simulink model "PV_microgrid"  (R2022b)
settings: Solver=FixedStepAuto  StartTime=0.0  StopTime=0.6  FixedStep=1e-6  RelTol=1e-3
model workspace (MAT data in the model file):
  C = 0.002
  D = 100
  GP = 1
  GQ = 1
  I1 = 100
  I2 = 50
  J = 3.5
  KQ = 0.06
  Kf = 120
  Kv = 577
  L = 2e-05
  LS = 0.003
  P1 = 0.2
  P2 = 6
  Pref = 500000
  Qref = 0
  Ts = 0.0001
  Ts_power = 1e-06
  Ug = 563.38264084
  fsw = 10000
  t0 = 0.5
  wn = 314.159265359
undefined symbols (not defined in the file): D1, Delta, DiscIntNeverNeededParam, Ion, Lithium, LL, LP, Ts_Power
libraries: spsSeriesRLCBranchLib x9, spsFirstOrderFilterLib x7, slpidlib x5, spsMeanLib x5, spsabctodq0Lib x4, spsStairGeneratorLib x4, spsThreePhaseVIMeasurementLib x3, spsThreePhaseTransformerTwoWindingsLib x2, spsThreePhaseParallelRLCLoadLib x2, spsThreePhasePISectionLineLib x2, spsBoostConverterLib x2, spsPowerPositiveSequenceLib x2
(part 1 of 2)
settings Model: SimulationMode=accelerator  Creator=刘明炜  LastModifiedBy=刘明炜

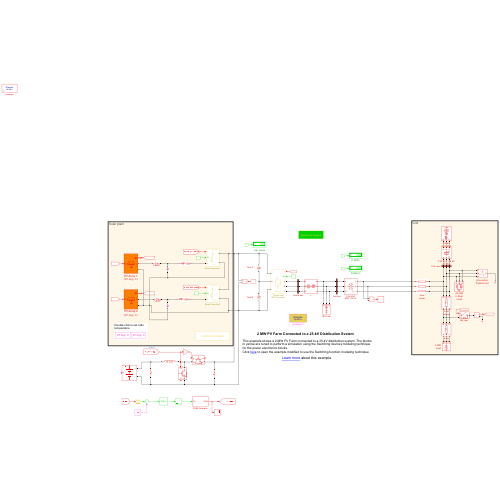
[thumbnail: Simulink's stored preview of the top-level diagram]
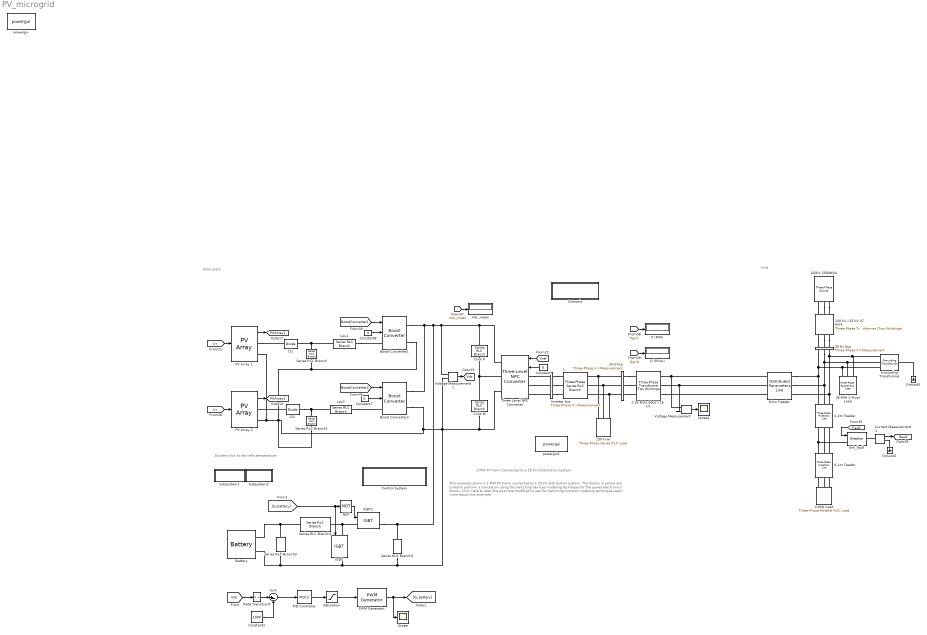
== system PV_microgrid ==
  note: Solar plant
  note: Double-click to set cells temperature
  note: This example shows a 2-MW PV Farm connected to a 25-kV distribution system. The blocks in yellow are tuned to perform a simulation using the Switching devices modeling technique for the power electronics blocks.
      | Click here to open the example modified to use the Switching function modeling technique
      |
      | Learn more about this example.
  note: 2 MW PV Farm Connected to a 25-kV Distribution System
  note: Grid
  120 kV / 25 kV 47 MVA : spsThreePhaseTransformerTwoWindingsLib/Three-Phase Transformer (Two Windings)  Winding1Connection=Yg  Winding2Connection=Delta (D1)  CoreType=Three single-phase transformers  SetSaturation=off  Hysteresis=off  DataFile='basic_model'  SetInitialFlux=off  Measurements=None  UNITS=pu  NominalPower=[47e6 50 ]  Winding1="[ 120e3  0.08/30   0.08 ]"  Winding2="[ 25e3 0.08/30  0.08]"  Rm=500  Lm=500  L0=0.5  Saturation="[ 0,0  ;  0.005,1.2  ;  1.0,1.4 ]"  InitialFluxes=[ 0.8 , -0.8 , 0.7 ]  BreakLoop=off  DiscreteSolver=Trapezoidal iterative  DataType=off  TransfoNumber=0
  120kV 2500MVA : spsThreePhaseSourceLib/Three-Phase Source  InternalConnection=Yg  VoltagePhases=off  Voltage=120e3*1.02  PhaseAngle=0  Voltage_phases=[25e3 25e3 25e3]/sqrt(3)  PhaseAngles_phases=[0 -120 +120]  Frequency=50  NonIdealSource=on  SpecifyImpedance=on  Resistance=0.8929  Inductance=16.58e-3  ShortCircuitLevel=2500e6  BaseVoltage=120e3  XRratio=7  BusType=swing  Pref=0  Qref=0  Prefabc=[10e3, 10e3, 10e3]  Qrefabc=[0, 0, 0]  Qmin=-inf  Qmax=inf
  150 kvar : spsThreePhaseSeriesRLCLoadLib/Three-Phase Series RLC Load  LConnTagsString=A|B|C  Configuration=Y (grounded)  NominalVoltage=500  Vabc=[1e3 1e3 1e3]  Vabcp=[1e3 1e3 1e3]  NominalFrequency=50  UnbalancedPower=off  ActivePower=150e3/50  InductivePower=0  CapacitivePower=150e3  Pabc=[10e3 9e3 11e3]  QLabc=[100 90 110]  QCabc=[100 90 110]  Pabcp=[10e3 9e3 11e3]  QLabcp=[100 90 110]  QCabcp=[100 90 110]  Measurements=None  LoadType=constant Z
  2-MW Load : spsThreePhaseParallelRLCLoadLib/Three-Phase Parallel RLC Load  LConnTagsString=A|B|C  Configuration=Y (grounded)  NominalVoltage=25e3  Vabc=[1e3 1e3 1e3]  Vabcp=[1e3 1e3 1e3]  NominalFrequency=50  UnbalancedPower=off  ActivePower=2e6  InductivePower=0  CapacitivePower=0  Pabc=[10e3 9e3 11e3]  QLabc=[100 90 110]  QCabc=[100 90 110]  Pabcp=[10e3 9e3 11e3]  QLabcp=[100 90 110]  QCabcp=[100 90 110]  Measurements=None  LoadType=constant Z
  2-km Feeder : spsThreePhasePISectionLineLib/Three-Phase PI Section Line  LConnTagsString=a|b|c  RConnTagsString=A|B|C  Length=2  Frequency=50  Resistances=[0.1153 0.413]  Inductances=[1.05e-3 3.32e-3]  Capacitances=[11.33e-009 5.01e-009]
  2.25-MVA 500V / 25 kV : spsThreePhaseTransformerTwoWindingsLib/Three-Phase Transformer (Two Windings)  Winding1Connection=Yg  Winding2Connection=Delta (D1)  CoreType=Three single-phase transformers  SetSaturation=off  Hysteresis=off  DataFile='hysteresis'  SetInitialFlux=off  Measurements=None  UNITS=pu  NominalPower=[2.25e6 , 50 ]  Winding1=[ 25e3 , 0.001 , 0.03 ]  Winding2=[500 , 0.001 , 0.03 ]  Rm=200  Lm=200  L0=0.5  Saturation=[ 0,0 ; 0.0024,1.2 ; 1.0,1.52 ]  InitialFluxes=[ 0.8 , -0.8 , 0.7 ]  BreakLoop=off  DiscreteSolver=Trapezoidal iterative  DataType=off  TransfoNumber=0
  25 Kv bus : spsThreePhaseVIMeasurementLib/Three-Phase V-I Measurement  VoltageMeasurement=phase-to-ground  SetLabelV=on  LabelV=Vabc25kV  Vpu=off  VpuLL=off  CurrentMeasurement=yes  SetLabelI=on  LabelI=Iabc25kV  Ipu=off  Pbase=100e6  Vbase=500e3  OutputType=Complex  PhasorSimulation=off  PSBequivalent=0
  30-MW 2-Mvar Load : spsThreePhaseParallelRLCLoadLib/Three-Phase Parallel RLC Load  LConnTagsString=A|B|C  Configuration=Y (grounded)  NominalVoltage=25e3  Vabc=[1e3 1e3 1e3]  Vabcp=[1e3 1e3 1e3]  NominalFrequency=50  UnbalancedPower=off  ActivePower=30e6  InductivePower=2e6  CapacitivePower=0  Pabc=[10e3 9e3 11e3]  QLabc=[100 90 110]  QCabc=[100 90 110]  Pabcp=[10e3 9e3 11e3]  QLabcp=[100 90 110]  QCabcp=[100 90 110]  Measurements=None  LoadType=constant Z
  6-km Feeder : spsThreePhasePISectionLineLib/Three-Phase PI Section Line  LConnTagsString=a|b|c  RConnTagsString=A|B|C  Length=6  Frequency=50  Resistances=[0.1153 0.413]  Inductances=[1.05e-3 3.32e-3]  Capacitances=[11.33e-009 5.01e-009]
  8-km Feeder : spsDistributedParametersLineLib/Distributed Parameters Line  Phases=3  Length=8  Frequency=50  Resistance=[0.1153 0.413]  Inductance=[1.05e-3 3.32e-3]  Capacitance=[11.33e-009 5.01e-009]  x1=[-3.3e-05 -0.02650333340574 -3248.46958209732 -24803.9467011853;-3.2e-05 -0.0265134078005961 -3240.67704414769 -24804.9660112382;-3.1e-05 -0.0265234795786837 -3232.88418635607 -24805.9828731392;-3e-05 -0.0265335487390089 -3225.09100949156 -24806.9972867877;-2.9e-05 -0.0265436152805778 -3217.29751432334 -24808.0092520839;-2.8e-05 -0.0265536792023969 -3209.50370162058 -24809.0187689276;-2.7e-05 -0.026563740503473 -3201.70957215251 -24810.0258372194;-2.6e-05 -0.0265737991828129 -3193.91512668837 -24811.0304568598;-2.5e-05 -0.0265838552394241 -3186.12036599744 -24812.0326277497;-2.4e-05 -0.0265939086723139 -3178.32529084904 -24813.0323497901;-2.3e-05 -0.0266039594804901 -3170.52990201251 -24814.0296228824;-2.2e-05 -0.0266140076629608 -3162.73420025723 -24815.0244469282;-2.1e-05 -0.0266240532187343 -3154.93818635259 -24816.0168218292;-2e-05 -0.026634096146819 -3147.14186106804 -24817.0067474876;-1.9e-05 -0.0266441364462239 -3139.34522517304 -24817.9942238056;-1.8e-05 -0.0266541741159579 -3131.54827943708 -24818.9792506858;-1.7e-05 -0.0266642091550304 -3123.75102462971 -24819.9618280309;-1.6e-05 -0.0266742415624509 -3115.95346152046 -24820.941955744;-1.5e-05 -0.0266842713372293 -3108.15559087894 -24821.9196337283;-1.4e-05 -0.0266942984783758 -3100.35741347476 -24822.8948618874;-1.3e-05 -0.0267043229849006 -3092.55893007757 -24823.867640125;-1.2e-05 -0.0267143448558144 -3084.76014145705 -24824.8379683451;-1.1e-05 -0.0267243640901281 -3076.96104838291 -24825.8058464519;-1e-05 -0.0267343806868528 -3069.16165162489 -24826.7712743499;-9e-06 -0.0267443946449998 -3061.36195195276 -24827.7342519438;-8e-06 -0.026754405963581 -3053.56195013632 -24828.6947791385;-7e-06 -0.0267644146416081 -3045.7616469454 -24829.6528558394;-6e-06 -0.0267744206780935 -3037.96104314985 -24830.6084819517;-5e-06 -0.0267844240720494 -3030.16013951957 -24831.5616573812;-4e-06 -0.0267944248224887 -3022.35893682447 -24832.5123820339;-3e-06 -0.0268044229284242 -3014.55743583451 -24833.4606558158;-2e-06 -0.0268144183888693 -3006.75563731965 -24834.4064786334;-1e-06 -0.0268244112028374 -2998.95354204991 -24835.3498503934]  x2=[-3.3e-05 -0.034117461108182 -3239.57935848846 -24789.857469648;-3.2e-05 -0.0341341498474203 -3231.79124723215 -24790.8739874484;-3.1e-05 -0.0341508352177531 -3224.00281701083 -24791.8880584878;-3e-05 -0.0341675172175336 -3216.21406859319 -24792.8996826658;-2.9e-05 -0.0341841958451153 -3208.42500274795 -24793.9088598828;-2.8e-05 -0.0342008710988521 -3200.63562024386 -24794.915590039;-2.7e-05 -0.0342175429770983 -3192.8459218497 -24795.9198730352;-2.6e-05 -0.0342342114782083 -3185.05590833427 -24796.9217087722;-2.5e-05 -0.0342508766005372 -3177.26558046643 -24797.9210971512;-2.4e-05 -0.0342675383424401 -3169.47493901505 -24798.9180380734;-2.3e-05 -0.0342841967022725 -3161.68398474904 -24799.9125314406;-2.2e-05 -0.0343008516783903 -3153.89271843732 -24800.9045771546;-2.1e-05 -0.0343175032691499 -3146.10114084888 -24801.8941751174;-2e-05 -0.0343341514729076 -3138.3092527527 -24802.8813252313;-1.9e-05 -0.0343507962880205 -3130.51705491781 -24803.8660273991;-1.8e-05 -0.0343674377128456 -3122.72454811328 -24804.8482815234;-1.7e-05 -0.0343840757457407 -3114.93173310819 -24805.8280875073;-1.6e-05 -0.0344007103850635 -3107.13861067166 -24806.8054452541;-1.5e-05 -0.0344173416291723 -3099.34518157285 -24807.7803546674;-1.4e-05 -0.0344339694764257 -3091.55144658093 -24808.7528156509;-1.3e-05 -0.0344505939251826 -3083.75740646512 -24809.7228281087;-1.2e-05 -0.0344672149738021 -3075.96306199465 -24810.690391945;-1.1e-05 -0.0344838326206439 -3068.1684139388 -24811.6555070644;-1e-05 -0.0345004468640679 -3060.37346306686 -24812.6181733715;-9e-06 -0.0345170577024343 -3052.57821014818 -24813.5783907714;-8e-06 -0.0345336651341036 -3044.7826559521 -24814.5361591693;-7e-06 -0.0345502691574369 -3036.98680124802 -24815.4914784706;-6e-06 -0.0345668697707953 -3029.19064680537 -24816.4443485812;-5e-06 -0.0345834669725404 -3021.39419339358 -24817.3947694068;-4e-06 -0.0346000607610342 -3013.59744178214 -24818.3427408538;-3e-06 -0.0346166511346389 -3005.80039274055 -24819.2882628286;-2e-06 -0.034633238091717 -2998.00304703837 -24820.2313352378;-1e-06 -0.0346498216306317 -2990.20540544514 -24821.1719579884]  x3=[-3.3e-05 0.0018330109232875 -5.20094376291286 -82.5841573333815;-3.2e-05 0.00183248031238211 -5.17499896715794 -82.5857871710294;-3.1e-05 0.00183194952061816 -5.1490536606511 -82.5874088577869;-3e-05 0.00183141854804805 -5.12310784595303 -82.5890223934939;-2.9e-05 0.00183088739472417 -5.0971615256245 -82.5906277779911;-2.8e-05 0.00183035606069894 -5.07121470222629 -82.5922250111202;-2.7e-05 0.00182982454602482 -5.04526737831925 -82.5938140927235;-2.6e-05 0.00182929285075425 -5.01931955646429 -82.5953950226442;-2.5e-05 0.00182876097493972 -4.99337123922235 -82.5969678007261;-2.4e-05 0.00182822891863372 -4.96742242915442 -82.5985324268142;-2.3e-05 0.00182769668188875 -4.94147312882156 -82.6000889007539;-2.2e-05 0.00182716426475736 -4.91552334078485 -82.6016372223917;-2.1e-05 0.00182663166729208 -4.88957306760544 -82.6031773915748;-2e-05 0.00182609888954548 -4.86362231184451 -82.6047094081511;-1.9e-05 0.00182556593157015 -4.8376710760633 -82.6062332719694;-1.8e-05 0.00182503279341869 -4.8117193628231 -82.6077489828793;-1.7e-05 0.00182449947514371 -4.78576717468524 -82.6092565407313;-1.6e-05 0.00182396597679785 -4.7598145142111 -82.6107559453766;-1.5e-05 0.00182343229843376 -4.73386138396209 -82.6122471966671;-1.4e-05 0.00182289844010412 -4.7079077864997 -82.6137302944556;-1.3e-05 0.00182236440186162 -4.68195372438544 -82.6152052385959;-1.2e-05 0.00182183018375897 -4.65599920018087 -82.6166720289423;-1.1e-05 0.00182129578584888 -4.6300442164476 -82.6181306653501;-1e-05 0.00182076120818411 -4.60408877574729 -82.6195811476753;-9e-06 0.0018202264508174 -4.57813288064163 -82.6210234757747;-8e-06 0.00181969151380155 -4.55217653369237 -82.6224576495061;-7e-06 0.00181915639718935 -4.52621973746131 -82.6238836687278;-6e-06 0.00181862110103361 -4.50026249451026 -82.6253015332991;-5e-06 0.00181808562538716 -4.47430480740111 -82.62671124308;-4e-06 0.00181754997030286 -4.44834667869578 -82.6281127979315;-3e-06 0.00181701413583357 -4.42238811095623 -82.6295061977153;-2e-06 0.00181647812203216 -4.39642910674448 -82.6308914422937;-1e-06 0.00181594192895156 -4.37046966862257 -82.63226853153]  x4=[-3.3e-05 -0.00190671760982347 -16.7682219944858 -79.8638556894328;-3.2e-05 -0.00190621989528535 -16.7431312365783 -79.8691196346485;-3.1e-05 -0.00190572199261087 -16.7180388261901 -79.8743756970982;-3e-05 -0.00190522390184916 -16.6929447657976 -79.8796238762631;-2.9e-05 -0.0019047256230494 -16.6678490578775 -79.8848641716251;-2.8e-05 -0.00190422715626075 -16.6427517049066 -79.8900965826671;-2.7e-05 -0.00190372850153242 -16.617652709362 -79.8953211088727;-2.6e-05 -0.00190322965891362 -16.5925520737209 -79.9005377497263;-2.5e-05 -0.00190273062845358 -16.5674498004605 -79.9057465047129;-2.4e-05 -0.00190223141020156 -16.5423458920583 -79.9109473733185;-2.3e-05 -0.00190173200420682 -16.5172403509921 -79.9161403550298;-2.2e-05 -0.00190123241051866 -16.4921331797396 -79.9213254493342;-2.1e-05 -0.00190073262918639 -16.4670243807788 -79.9265026557201;-2e-05 -0.00190023266025932 -16.4419139565879 -79.9316719736764;-1.9e-05 -0.00189973250378681 -16.4168019096451 -79.936833402693;-1.8e-05 -0.00189923215981822 -16.3916882424289 -79.9419869422604;-1.7e-05 -0.00189873162840292 -16.3665729574179 -79.94713259187;-1.6e-05 -0.00189823090959033 -16.341456057091 -79.9522703510139;-1.5e-05 -0.00189773000342986 -16.316337543927 -79.9574002191851;-1.4e-05 -0.00189722890997095 -16.2912174204051 -79.9625221958773;-1.3e-05 -0.00189672762926305 -16.2660956890044 -79.967636280585;-1.2e-05 -0.00189622616135564 -16.2409723522045 -79.9727424728033;-1.1e-05 -0.00189572450629821 -16.2158474124848 -79.9778407720284;-1e-05 -0.00189522266414027 -16.1907208723252 -79.9829311777571;-9e-06 -0.00189472063493136 -16.1655927342055 -79.988013689487;-8e-06 -0.00189421841872101 -16.1404630006058 -79.9930883067164;-7e-06 -0.0018937160155588 -16.1153316740062 -79.9981550289445;-6e-06 -0.00189321342549432 -16.0901987568872 -80.0032138556712;-5e-06 -0.00189271064857716 -16.0650642517292 -80.0082647863973;-4e-06 -0.00189220768485695 -16.0399281610129 -80.0133078206242;-3e-06 -0.00189170453438332 -16.0147904872192 -80.0183429578543;-2e-06 -0.00189120119720595 -15.989651232829 -80.0233701975905;-1e-06 -0.0018906976733745 -15.9645104003235 -80.0283895393367]  x5=3.26270562570392e-05  V1=ones(3,3)  V2=ones(3,3)  I1=ones(3,3)  I2=ones(3,3)  nHarmo=1  Measurements=None  Decoupling=off  VsMag0=0  VrMag0=0  VsAngle0=0  VrAngle0=0  IsMag0=0  IrMag0=0  IsAngle0=0  IrAngle0=0
      settings: LibrarySourceBlock=sps_lib/Power Grid Elements/Distributed Parameters Line
  Battery : spsBatteryLib/Battery  BatType=Lithium-Ion  ShowTempParam=off  ThermalPreset=no  ShowAgeParam=off  NomV=150  NomQ=15000  SOC=80  Batt_Tr=30  PresetModel=on  MaxQ=15000  MinV=112.5  FullV=174.5981  Dis_rate=6521.7391  R=0.0001  Normal_OP=13565.2174  expZone="[162.0579      736.9565]"  current=[6.5 13 32.5]  Units=Time  Tci=20  NomT=20  T2=-30  MaxQ2=4.8  FullV2=7.1  Normal_OP2=5.655  expZone2="[6.58           1]"  Rca=0.6  ti=2000  Dp=0  Neq0=0  Tsim=1e6  Ta1=25  Qeol=5.4*0.9  Reol=0.013333*1.2  Char_age=[2.3478, 3]  Dis_age=[2.3478, 10]  N1=1500  N2=10500  N3=1000  N4=1400  Ta2=45  N5=950
  Boost Converter1 : spsBoostConverterLib/Boost Converter  ModelType=Switching devices  Ron=1e-4  Rs=1e6  Cs=inf  Vforward=[0,0]  Ron_Diode=1e-4  Rs_Diode=1e6  Cs_Diode=inf  Vf_Diode=0  Rs_CurrentSource=inf  Ron_ACsource=1e-3
      settings: LibrarySourceBlock=sps_lib/Power Electronics/Boost Converter
  Boost Converter2 : spsBoostConverterLib/Boost Converter  ModelType=Switching devices  Ron=1e-4  Rs=1e6  Cs=inf  Vforward=[0,0]  Ron_Diode=1e-4  Rs_Diode=1e6  Cs_Diode=inf  Vf_Diode=0  Rs_CurrentSource=inf  Ron_ACsource=1e-3
      settings: LibrarySourceBlock=sps_lib/Power Electronics/Boost Converter
  Brk_fault : spsBreakerLib/Breaker  InitialState=0  SwitchingTimes="[30/60  42/60]*999"  External=on  BreakerResistance=0.2  SnubberResistance=1e6  SnubberCapacitance=inf  Measurements=None  MoreParameters=on  NoBreakLoop=off
  Clink M : spsSeriesRLCBranchLib/Series RLC Branch  LConnTagsString=__new0  RConnTagsString=__new0  BranchType=C  Resistance=1e-6  Inductance=1e-3  SetiL0=off  InitialCurrent=0  Capacitance=150e-3  Setx0=on  InitialVoltage=500  Measurements=None
  Clink P : spsSeriesRLCBranchLib/Series RLC Branch  LConnTagsString=__new0  RConnTagsString=__new0  BranchType=C  Resistance=1e-6  Inductance=1e-3  SetiL0=off  InitialCurrent=0  Capacitance=150e-3  Setx0=on  InitialVoltage=500  Measurements=None
  Constant : Constant  Value=0  SampleTime=Ts
  Constant1 : Constant  Value=1000
  Constant7 : Constant  Value=0  SampleTime=Ts
  Constant8 : Constant  Value=0  SampleTime=Ts
  Control System : Subsystem
      mask Display: disp('CONTROL SYSTEM')
  Current Measurement1 : spsCurrentMeasurementLib/Current Measurement  PhasorSimulation=off  OutputType=Complex  PSBequivalent=0
  D1 : spsDiodeLib/Diode  Ron=1e-4  Lon=0  Vf=0  IC=0  UseSnubber=0  Rs=1e6  Cs=inf  Measurements=off
  D2 : spsDiodeLib/Diode  Ron=1e-4  Lon=0  Vf=0  IC=0  UseSnubber=0  Rs=1e6  Cs=inf  Measurements=off
  Grid bus : spsThreePhaseVIMeasurementLib/Three-Phase V-I Measurement  VoltageMeasurement=phase-to-ground  SetLabelV=on  LabelV=Ugrid  Vpu=off  VpuLL=off  CurrentMeasurement=yes  SetLabelI=on  LabelI=Igrid  Ipu=off  Pbase=100e6  Vbase=500e3  OutputType=Magnitude  PhasorSimulation=off  PSBequivalent=0
  Ground2 : spsGroundLib/Ground  LConnTagsString=a
  Ground3 : spsGroundLib/Ground  LConnTagsString=a
  Grounding Transformer : spsGroundingTransformerLib/Grounding Transformer   UNITS=SI  NominalPower="[3e6   50]"  NominalVoltage=25e3  ZeroSequenceImpedance_pu=[0.0012 0.036]  MagnetizationBranch_pu=[500 500]  ZeroSequenceImpedance_SI=[0.25 7.5]  MagnetizationBranch_SI=[1.0417e+05 1.0417e+05]  Measurements=None
      settings: LibrarySourceBlock=|
      | sps_lib/Power Grid Elements/Grounding
      | Transformer
  IGBT : spsIGBTLib/IGBT  Ron=0.001  Lon=0  Vf=1  Tf=1e-6  Tt=2e-6  IC=0  Rs=1e5  Cs=inf  Measurements=on
  IGBT1 : spsIGBTLib/IGBT  Ron=0.001  Lon=0  Vf=1  Tf=1e-6  Tt=2e-6  IC=0  Rs=1e5  Cs=inf  Measurements=on
  Inverter bus : spsThreePhaseVIMeasurementLib/Three-Phase V-I Measurement  VoltageMeasurement=phase-to-phase  SetLabelV=on  LabelV=Vinv  Vpu=off  VpuLL=off  CurrentMeasurement=yes  SetLabelI=on  LabelI=ILabc  Ipu=off  Pbase=100e6  Vbase=500e3  OutputType=Magnitude  PhasorSimulation=off  PSBequivalent=0
  L : spsThreePhaseSeriesRLCBranchLib/Three-Phase Series RLC Branch  LConnTagsString=A|B|C  RConnTagsString=A|B|C  BranchType=RL  Resistance=1e-3  Inductance=44.2e-6  Capacitance=inf  Measurements=None
  Lpv1 : spsSeriesRLCBranchLib/Series RLC Branch  LConnTagsString=__new0  RConnTagsString=__new0  BranchType=RL  Resistance=1e-3  Inductance=1e-3  SetiL0=off  InitialCurrent=0  Capacitance=120e-3  Setx0=off  InitialVoltage=0  Measurements=None
  Lpv2 : spsSeriesRLCBranchLib/Series RLC Branch  LConnTagsString=__new0  RConnTagsString=__new0  BranchType=RL  Resistance=1e-3  Inductance=1e-3  SetiL0=off  InitialCurrent=0  Capacitance=120e-3  Setx0=off  InitialVoltage=0  Measurements=None
  NOT : Logic  Operator=NOT  IconShape=distinctive  AllPortsSameDT=off  OutDataTypeStr=boolean
  P (MW) : Display
      settings: Format=bank  Decimation=200
  PID Controller : slpidlib/PID Controller  Controller=PID  Form=Parallel  TimeDomain=Discrete-time  UseExternalTs=off  SampleTime=-1  IntegratorMethod=Forward Euler  FilterMethod=Forward Euler  ControllerParametersSource=internal  P=1  I=1  UseKiTs=off  D=0  N=100  UseFilter=on  TunerSelectOption=Transfer Function Based (PID Tuner App)  InitialConditionSource=internal  InitialConditionForIntegrator=0  InitialConditionForFilter=0  DifferentiatorICPrevScaledInput=0  ExternalReset=none  TrackingMode=off  Kt=1  LimitOutput=off  SatLimitsSource=internal  UpperSaturationLimit=0.99  LowerSaturationLimit=0.1  LinearizeAsGain=on  AntiWindupMode=none  Kb=1  LimitIntegrator=off  UpperIntegratorSaturationLimit=inf  LowerIntegratorSaturationLimit=-inf  POutMin=[]  POutMax=[]  IOutMin=[]  IOutMax=[]  DOutMin=[]  DOutMax=[]  NOutMin=[]  NOutMax=[]  SumOutMin=[]  SumOutMax=[]  SaturationOutMin=[]  SaturationOutMax=[]  PParamMin=[]  PParamMax=[]  IParamMin=[]  IParamMax=[]  DParamMin=[]  DParamMax=[]  NParamMin=[]  NParamMax=[]  KbParamMin=[]  KbParamMax=[]  KtParamMin=[]  KtParamMax=[]  KbOutMin=[]  KbOutMax=[]  KtOutMin=[]  KtOutMax=[]  IntegratorOutMin=[]  IntegratorOutMax=[]  FilterOutMin=[]  FilterOutMax=[]  SumI1OutMin=[]  SumI1OutMax=[]  SumI2OutMin=[]  SumI2OutMax=[]  SumI3OutMin=[]  SumI3OutMax=[]  SumI4OutMin=[]  SumI4OutMax=[]  SumDOutMin=[]  SumDOutMax=[]  DifferentiatorOutMin=[]  DifferentiatorOutMax=[]  FilterDiffOutCoefMin=[]  FilterDiffOutCoefMax=[]  ReciprocalOutMin=[]  ReciprocalOutMax=[]  SumDenOutMin=[]  SumDenOutMax=[]  SumNumOutMin=[]  SumNumOutMax=[]  DivideOutMin=[]  DivideOutMax=[]  UdiffTsProdOutMin=[]  UdiffTsProdOutMax=[]  NTsProdOutMin=[]  NTsProdOutMax=[]  UintegralTsProdOutMin=[]  UintegralTsProdOutMax=[]  UngainTsProdOutMin=[]  UngainTsProdOutMax=[]  ClampingZeroOutDataTypeStr=Inherit: Inherit via back propagation  ClampingZeroOutMin=[]  ClampingZeroOutMax=[]  FilterDenConstantOutDataTypeStr=Inherit: Inherit via back propagation  FilterDenConstantOutMin=[]  FilterDenConstantOutMax=[]  PCopyOutDataTypeStr=Inherit: Inherit via back propagation  PCopyOutMin=[]  PCopyOutMax=[]  NCopyOutDataTypeStr=Inherit: Inherit via back propagation  NCopyOutMin=[]  NCopyOutMax=[]  IntegratorContinuousStateAttributes=''  IntegratorStateMustResolveToSignalObject=off  IntegratorRTWStateStorageClass=Auto  FilterContinuousStateAttributes=''  FilterStateMustResolveToSignalObject=off  FilterRTWStateStorageClass=Auto  ParallelPVariant=InternalParameters  IdealPVariant=Disabled  IVariant=InternalParameters  DVariant=InternalParameters  IntegratorVariant=Discrete  SatVariant=Disabled  AWVariant=Passthrough  PCopyVariant=Disabled  TRVariant=Disabled  FdbkBlocksVariant=Forward  IdealPFdbkVariant=Disabled  SatFdbkVariant=Disabled  DerivativeFilterVariant=ForwardEulerFilter  NVariant=InternalParameters  NCopyVariant=Disabled  FilterICVariant=InternalICsFilter  IntegratorICVariant=InternalICs  ExternalResetVariant=Disabled  TRSumVariant=Passthrough  SumFdbkVariant=Disabled  SumVariant=Sum_PID  TsampFilterVariant=InternalTs  TsampNgainVariant=Passthrough  TsampIntegralVariant=Passthrough  ExternalSaturationOutDataTypeStr=Inherit: Same as second input
  PV Array 1 : spsPVArrayLib/PV Array  Npar=282  Nser=15  PlotType=array @ 1000 W/m2 & specified temperatures  S_vec=[ 1000 250]  Temp_C_vec="[ 45 25  ]"  ModuleName=User-defined  PlotWhenSelected=off  Pm=355.012  Ncell=83  Voc=51.9  Isc=8.68  Vm=43.4  Im=8.18  beta_Voc_pc=-0.304  alpha_Isc_pc=0.017  beta_Voc=-0.15778  alpha_Isc=0.0014756  IL=8.6865  I0=3.3093e-11  nI=0.92618  Rsh=389.4331  Rs=0.29289  RobustModel=on  RobustCellTemperature=25  BAL=on  Tc=1e-6  Tfilter=5e-5
      settings: AttributesFormatString=(%<RobustCellTemperature> deg. C)
  PV Array 2 : spsPVArrayLib/PV Array  Npar=122  Nser=14  PlotType=array @ 1000 W/m2 & specified temperatures  S_vec=[ 1000 250]  Temp_C_vec="[ 45 25  ]"  ModuleName=User-defined  PlotWhenSelected=off  Pm=293.664  Ncell=60  Voc=39.5  Isc=9.60  Vm=32.2  Im=9.12  beta_Voc_pc=-0.300  alpha_Isc_pc=0.03  beta_Voc=-0.1185  alpha_Isc=0.00288  IL=9.6627  I0=3.1923e-11  nI=0.96973  Rsh=336.4947  Rs=0.3029  RobustModel=on  RobustCellTemperature=25  BAL=on  Tc=1e-6  Tfilter=5e-5
      settings: AttributesFormatString=(%<RobustCellTemperature> deg. C)
  PWM Generator : eePwmGenerator/PWM Generator  CarrCount=Up  Tper=fsw  Tdelay=0  Ts=Ts_power
  Q (Mvar) : Display
      settings: Format=bank  Decimation=200
  Rate Transition5 : RateTransition  OutPortSampleTime=Ts
  Saturation : Saturate  UpperLimit=0.99  LowerLimit=0.1
  Scenario : Subsystem
      mask Display: disp('Scenario & Scopes')
  Scope : Scope
  Scope1 : Scope
  Series RLC Branch : spsSeriesRLCBranchLib/Series RLC Branch  LConnTagsString=__new0  RConnTagsString=__new0  BranchType=C  Resistance=1  Inductance=1e-3  SetiL0=off  InitialCurrent=0  Capacitance=200e-6  Setx0=on  InitialVoltage=650  Measurements=None
  Series RLC Branch1 : spsSeriesRLCBranchLib/Series RLC Branch  LConnTagsString=__new0  RConnTagsString=__new0  BranchType=C  Resistance=1  Inductance=1e-3  SetiL0=off  InitialCurrent=0  Capacitance=200e-6  Setx0=on  InitialVoltage=450  Measurements=None
  Series RLC Branch2 : spsSeriesRLCBranchLib/Series RLC Branch  LConnTagsString=__new0  RConnTagsString=__new0  BranchType=L  Resistance=1  Inductance=1e-3  SetiL0=off  InitialCurrent=0  Capacitance=1e-6  Setx0=off  InitialVoltage=0  Measurements=None
  Series RLC Branch3 : spsSeriesRLCBranchLib/Series RLC Branch  LConnTagsString=__new0  RConnTagsString=__new0  BranchType=C  Resistance=1  Inductance=1e-3  SetiL0=off  InitialCurrent=0  Capacitance=1e-6  Setx0=off  InitialVoltage=0  Measurements=None
  Series RLC Branch5 : spsSeriesRLCBranchLib/Series RLC Branch  LConnTagsString=__new0  RConnTagsString=__new0  BranchType=C  Resistance=1  Inductance=1e-3  SetiL0=off  InitialCurrent=0  Capacitance=1e-6  Setx0=off  InitialVoltage=0  Measurements=None
  Subsystem1 : Subsystem
      settings: OpenFcn=|
      | SystemName1=gcs;
      | BlockName1=[SystemName1, '/', 'PV Array 1'];
      | set_param(BlockName1,'RobustCellTemperature','25');
      | set_param(BlockName1,'ForegroundColor','black');
      | BlockName2=[SystemName1, '/', 'PV Array 2'];
      | set_param(BlockName2,'RobustCellTemperature','25');
      | set_param(BlockName2,'ForegroundColor','black');
      mask Display: disp('25 deg. C')
  Subsystem2 : Subsystem
      settings: OpenFcn=|
      | SystemName1=gcs;
      | BlockName1=[SystemName1, '/', 'PV Array 1'];
      | set_param(BlockName1,'RobustCellTemperature','45');
      | set_param(BlockName1,'ForegroundColor','red');
      | BlockName2=[SystemName1, '/', 'PV Array 2'];
      | set_param(BlockName2,'RobustCellTemperature','45');
      | set_param(BlockName2,'ForegroundColor','red');
      mask Display: disp('45 deg. C')
  Sum : Sum  Inputs=|+-
  Three-Level NPC Converter : spsThreeLevelNPCConverterLib/Three-Level NPC Converter  ModelType=Switching devices  Ron=1e-4/2  Rs=1e6  Cs=inf  Vforward=[0,0]  Ron_Diode=1e-4  Rs_Diode=1e6  Cs_Diode=inf  Vf_Diode=0  Rs_CurrentSource=inf  Ron_ACsource=1e-3
      settings: LibrarySourceBlock=|
      | sps_lib/Power Electronics/Three-Level
      | NPC Converter
  Vdc_mean : Display
      settings: Decimation=200
  Voltage Measurement : spsVoltageMeasurementLib/Voltage Measurement  PhasorSimulation=off  OutputType=Complex  PSBequivalent=0
  Voltage Measurement1 : spsVoltageMeasurementLib/Voltage Measurement  PhasorSimulation=off  OutputType=Complex  PSBequivalent=0
  powergui : spspowerguiLib/powergui  Priority=1  SimulationMode=Discrete  SampleTime=1e-6  frequency=60  Iterations=50  frequencyindice=0  Pbase=100e6  ErrMax=1e-4  UnitsV=kV  UnitsW=MW  buscounter=0  FunctionMessages=off  echomessages=off  EnableUseOfTLC=off  CurrentSourceSwitches=off  DisableSnubberDevices=off  DisableRonSwitches=off  DisableVfSwitches=off  DisplayEquations=off  AutomaticDiscreteSolvers=off  SolverType=Tustin/Backward Euler (TBE)  Interpol=off  ExternalGateDelay=off  methode=off  Ts=100  x0status=blocks  SPID=on  SwTol=0  HookPort=off  NonlinearTolerance=1e-4  nMaxIteration=100  ContinueOnMaxIteration=off  RestoreLinks=warning  ResistiveCurrentMeasurement=off  Frange=[0:2:500]  Ylog=off  Xlog=on  ShowGrid=off  save=off  variable=ZData  structure=0  ZoomFFT=off  StartTime=0.0  cycles=1  DisplayStyle=1  fundamental=60  FreqAxis=off  MaxFrequency=1000  frequencyindicesteady=1  RmsSteady=1  display=off
  powergui1 : spspowerguiLib/powergui  Priority=2  SimulationMode=Discrete  SampleTime=Ts_Power  frequency=60  Iterations=50  frequencyindice=0  Pbase=100e6  ErrMax=1e-4  UnitsV=kV  UnitsW=MW  buscounter=0  FunctionMessages=off  echomessages=off  EnableUseOfTLC=off  CurrentSourceSwitches=off  DisableSnubberDevices=off  DisableRonSwitches=off  DisableVfSwitches=off  DisplayEquations=off  AutomaticDiscreteSolvers=off  SolverType=Tustin/Backward Euler (TBE)  Interpol=off  ExternalGateDelay=off  methode=off  Ts=0  x0status=blocks  SPID=off  SwTol=0  HookPort=off  NonlinearTolerance=1e-4  nMaxIteration=100  ContinueOnMaxIteration=on  RestoreLinks=warning  ResistiveCurrentMeasurement=off  Frange=[0:2:500]  Ylog=off  Xlog=off  ShowGrid=off  save=off  variable=ZData  structure=Scope_VIgrid  ZoomFFT=off  StartTime=0.18  cycles=1  DisplayStyle=1  fundamental=60  FreqAxis=on  MaxFrequency=3500  frequencyindicesteady=1  RmsSteady=1  display=off
  tag scope: Ifault=global, PVArray1=global, PVArray2=global, Vdc=global
  wires:
  [Fault] -> Brk_fault/1
  PV Array 1/1 -> [PVArray1]
  [Irr] -> PV Array 2/1
  Constant8/1 -> Boost Converter1/2
  Voltage Measurement1/1 -> [Vdc]
  [Vref] -> Three-Level NPC Converter/1
  [Qgrid] -> Q (Mvar)/1
  [BoostConverter1] -> Boost Converter1/1
  Constant7/1 -> Boost Converter2/2
  [Vdc_mean] -> Vdc_mean/1
  [Pgrid] -> P (MW)/1
  [Irr] -> PV Array 1/1
  Current Measurement1/1 -> [Ifault]
  Constant/1 -> Three-Level NPC Converter/2
  PV Array 2/1 -> [PVArray2]
  [BoostConverter2] -> Boost Converter2/1
  Sum/1 -> PID Controller/1
  Constant1/1 -> Sum/2
  PID Controller/1 -> Saturation/1
  [G_battery] -> IGBT/1, NOT/1
  NOT/1 -> IGBT1/1
  [Vdc] -> Rate Transition5/1
  Rate Transition5/1 -> Sum/1
  PWM Generator/1 -> Scope/1, [G_battery]
  Saturation/1 -> PWM Generator/1
  Voltage Measurement/1 -> Scope1/1
  connections:
  2-km Feeder/RConn1 -- 6-km Feeder/LConn1 -- Brk_fault/LConn1
  IGBT/RConn1 -- Clink M/RConn1 -- Three-Level NPC Converter/RConn3 -- Boost Converter2/RConn2 -- Series RLC Branch1/RConn1 -- PV Array 2/RConn2 -- PV Array 1/RConn2 -- Series RLC Branch/RConn1 -- Boost Converter1/RConn2 -- Voltage Measurement1/LConn2 -- Series RLC Branch5/RConn1 -- Series RLC Branch3/RConn1 -- Battery/LConn2
  150 kvar/LConn1 -- Grid bus/LConn1 -- L/RConn1
  30-MW 2-Mvar Load/LConn1 -- Grounding Transformer/LConn1 -- 25 Kv bus/RConn1 -- 8-km Feeder/RConn1 -- 2-km Feeder/LConn1
  Grounding Transformer/LConn3 -- 30-MW 2-Mvar Load/LConn3 -- 25 Kv bus/RConn3 -- 8-km Feeder/RConn3 -- 2-km Feeder/LConn3
  Series RLC Branch1/LConn1 -- Lpv2/RConn1 -- D2/RConn1
  8-km Feeder/RConn2 -- 25 Kv bus/RConn2 -- 30-MW 2-Mvar Load/LConn2 -- Grounding Transformer/LConn2 -- 2-km Feeder/LConn2
  150 kvar/LConn3 -- Grid bus/LConn3 -- L/RConn3
  150 kvar/LConn2 -- L/RConn2 -- Grid bus/LConn2
  IGBT1/RConn1 -- Voltage Measurement1/LConn1 -- Three-Level NPC Converter/RConn1 -- Clink P/LConn1 -- Boost Converter1/RConn1 -- Boost Converter2/RConn1 -- Series RLC Branch5/LConn1
  Three-Level NPC Converter/RConn2 -- Clink M/LConn1 -- Clink P/RConn1
  Series RLC Branch/LConn1 -- Lpv1/RConn1 -- D1/RConn1
  Inverter bus/RConn2 -- L/LConn2
  Current Measurement1/LConn1 -- Brk_fault/RConn1
  2-MW Load/LConn3 -- 6-km Feeder/RConn3
  2-MW Load/LConn1 -- 6-km Feeder/RConn1
  Inverter bus/RConn3 -- L/LConn3
  120 kV / 25 kV 47 MVA/RConn2 -- 25 Kv bus/LConn2
  120kV 2500MVA/RConn3 -- 120 kV / 25 kV 47 MVA/LConn3
  PV Array 1/RConn1 -- D1/LConn1
  8-km Feeder/LConn1 -- Voltage Measurement/LConn1 -- 2.25-MVA 500V / 25 kV/LConn1
  Inverter bus/RConn1 -- L/LConn1
  Current Measurement1/RConn1 -- Ground2/LConn1
  Three-Level NPC Converter/LConn2 -- Inverter bus/LConn2
  Three-Level NPC Converter/LConn3 -- Inverter bus/LConn3
  Lpv1/LConn1 -- Boost Converter1/LConn1
  6-km Feeder/LConn3 -- 2-km Feeder/RConn3
  Three-Level NPC Converter/LConn1 -- Inverter bus/LConn1
  120kV 2500MVA/RConn1 -- 120 kV / 25 kV 47 MVA/LConn1
  2-MW Load/LConn2 -- 6-km Feeder/RConn2
  D2/LConn1 -- PV Array 2/RConn1
  6-km Feeder/LConn2 -- 2-km Feeder/RConn2
  Ground3/LConn1 -- Grounding Transformer/RConn1
  120 kV / 25 kV 47 MVA/RConn3 -- 25 Kv bus/LConn3
  120kV 2500MVA/RConn2 -- 120 kV / 25 kV 47 MVA/LConn2
  120 kV / 25 kV 47 MVA/RConn1 -- 25 Kv bus/LConn1
  Lpv2/LConn1 -- Boost Converter2/LConn1
  2.25-MVA 500V / 25 kV/LConn2 -- Voltage Measurement/LConn2 -- 8-km Feeder/LConn2
  2.25-MVA 500V / 25 kV/LConn3 -- 8-km Feeder/LConn3
  Series RLC Branch2/LConn1 -- Series RLC Branch3/LConn1 -- Battery/LConn1
  Series RLC Branch2/RConn1 -- IGBT1/LConn1 -- IGBT/LConn1
  Grid bus/RConn1 -- 2.25-MVA 500V / 25 kV/RConn1
  Grid bus/RConn2 -- 2.25-MVA 500V / 25 kV/RConn2
  Grid bus/RConn3 -- 2.25-MVA 500V / 25 kV/RConn3

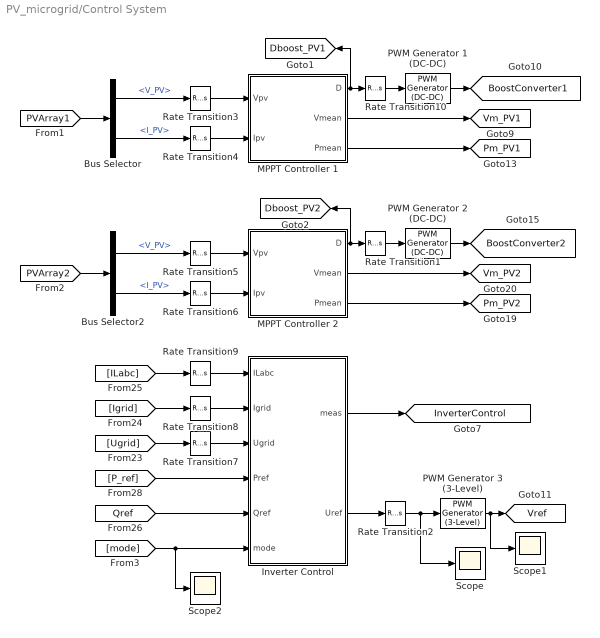
== system PV_microgrid/Control System ==
  Bus Selector : BusSelector  OutputSignals=V_PV,I_PV
  Bus Selector2 : BusSelector  OutputSignals=V_PV,I_PV
  Inverter Control : Subsystem  mask(Inverter Control){Pnom=2.25e6, Fnom=50, Vnom_prim=25e3, Vnom_sec=500, Vnom_dc=1000, Kp_Preg=1, Ki_Preg=75, Kp_VDCreg=10, Ki_VDCreg=500, Kp_Ireg=0.3, Ki_Ireg=20, RLff=[0.004, 0.21], Ts=Ts}
      mask prompts: Pnom "Power (VA)"; Fnom "Frequency (Hz)"; Vnom_prim "Primary voltage (Vrms)"; Vnom_sec "Secondary voltage (Vrms)"; Vnom_dc "DC voltage (V)"; Kp_Preg "Proportional gain"; Ki_Preg "Integral gain"; Kp_VDCreg "Proportional gain"; Ki_VDCreg "Integral gain"; Kp_Ireg "Proportional gain"; Ki_Ireg "Integral gain"; RLff "Feedforward Values [Rff Lff] (pu)"; Ts "Control sample time:"
      mask help: Control system for a 2-MW, 1-Mvar, 25-kV, Grid-Connected Inverter
      mask init:
      | Rff=RLff(1);
      | Lff=RLff(2);
      | Limits_Ireg=[1.5, -1.5];
      | Limits_VDCreg=[1.5, -1.5];
      | Limits_Preg=[1.5, -1.5];
      | Limits_Qreg=[1.5, -1.5];
      mask DialogControl Container4 Prompt: Nominal Values:
      mask DialogControl Container16 Prompt: Power regulators
      mask DialogControl Container8 Prompt: Voltage regulator:
      mask DialogControl Container6 Prompt: Current regulators:
      mask DialogControl Ts1 Prompt: Sample time (s)
  MPPT Controller 1 : Subsystem  mask(MPPT Controller - Perturb and Observe algorithm (PandO)){Dinit=0.35, Dlimits=[0.8, 0.3], deltaD=60e-6, Fc=1000, Ts=Ts}
      mask prompts: Dinit "Duty cycle (D) initial value"; Dlimits "D limits [Upper, Lower]"; deltaD "Increment value for PandO algorithm"; Fc "Measurement filter cutoff frequency (Hz)"; Ts "Sample time (s)"
      mask init:
      | Dmax=Dlimits(1);
      | Dmin=Dlimits(2);
  MPPT Controller 2 : Subsystem  mask(MPPT Controller - Perturb and Observe algorithm (PandO)){Dinit=0.55, Dlimits=[0.8, 0.47], deltaD=60e-6, Fc=1000, Ts=Ts}
      mask prompts: Dinit "Duty cycle (D) initial value"; Dlimits "D limits [Upper, Lower]"; deltaD "Increment value for PandO algorithm"; Fc "Measurement filter cutoff frequency (Hz)"; Ts "Sample time (s)"
      mask init:
      | Dmax=Dlimits(1);
      | Dmin=Dlimits(2);
  PWM Generator 1 (DC-DC) : spsPWMGeneratorDCDCLib/PWM Generator (DC-DC)  Fsw=5000  Ts=Ts_Power
  PWM Generator 2 (DC-DC) : spsPWMGeneratorDCDCLib/PWM Generator (DC-DC)  Fsw=5000  Ts=Ts_Power
  PWM Generator 3 (3-Level) : spsPWMGenerator3LevelLib/PWM Generator (3-Level)  ModulatorType=Three-phase bridge (12 pulses)  ModulatorMode=Unsynchronized  nF=27  Fc=39*60  ModulatingSignals=off  m=0.8  Freq=60  Phase=0  Ts=Ts_Power
      settings: LibrarySourceBlock=|
      | sps_lib/Power Electronics/Power Electronics Control/PWM Generator
      | (3-Level)
  Rate Transition1 : RateTransition  OutPortSampleTime=Ts_Power
  Rate Transition10 : RateTransition  OutPortSampleTime=Ts_Power
  Rate Transition2 : RateTransition  OutPortSampleTime=Ts_Power
  Rate Transition{3..9} (7 alike) : RateTransition  OutPortSampleTime=Ts
  Scope : Scope
  Scope1 : Scope
  Scope2 : Scope
  tag scope: BoostConverter1=global, BoostConverter2=global, Dboost_PV1=global, Dboost_PV2=global, InverterControl=global, Pm_PV1=global, Pm_PV2=global, Vm_PV1=global, Vm_PV2=global, Vref=global
  wires:
  Inverter Control/2(Uref) -> Rate Transition2/1
  MPPT Controller 2/2(Vmean) -> [Vm_PV2]
  [Ugrid] -> Rate Transition7/1
  [P_ref] -> Inverter Control/4(Pref)
  Bus Selector2/1 -> Rate Transition5/1  "<V_PV>"
  Rate Transition3/1 -> MPPT Controller 1/1(Vpv)
  Rate Transition2/1 -> Scope/1, PWM Generator 3 (3-Level)/1
  Rate Transition4/1 -> MPPT Controller 1/2(Ipv)
  [Igrid] -> Rate Transition8/1
  Bus Selector/2 -> Rate Transition4/1  "<I_PV>"
  MPPT Controller 2/3(Pmean) -> [Pm_PV2]
  [Qref] -> Inverter Control/5(Qref)
  [ILabc] -> Rate Transition9/1
  MPPT Controller 1/1(D) -> [Dboost_PV1], Rate Transition10/1
  Bus Selector/1 -> Rate Transition3/1  "<V_PV>"
  Bus Selector2/2 -> Rate Transition6/1  "<I_PV>"
  Rate Transition1/1 -> PWM Generator 2 (DC-DC)/1
  Rate Transition6/1 -> MPPT Controller 2/2(Ipv)
  Rate Transition8/1 -> Inverter Control/2(Igrid)
  Rate Transition7/1 -> Inverter Control/3(Ugrid)
  MPPT Controller 1/3(Pmean) -> [Pm_PV1]
  MPPT Controller 1/2(Vmean) -> [Vm_PV1]
  Rate Transition9/1 -> Inverter Control/1(ILabc)
  Rate Transition10/1 -> PWM Generator 1 (DC-DC)/1
  MPPT Controller 2/1(D) -> [Dboost_PV2], Rate Transition1/1
  Rate Transition5/1 -> MPPT Controller 2/1(Vpv)
  PWM Generator 1 (DC-DC)/1 -> [BoostConverter1]
  PWM Generator 2 (DC-DC)/1 -> [BoostConverter2]
  Inverter Control/1(meas) -> [InverterControl]
  PWM Generator 3 (3-Level)/1 -> Scope1/1, [Vref]
  [PVArray1] -> Bus Selector/1
  [PVArray2] -> Bus Selector2/1
  [mode] -> Scope2/1, Inverter Control/6(mode)

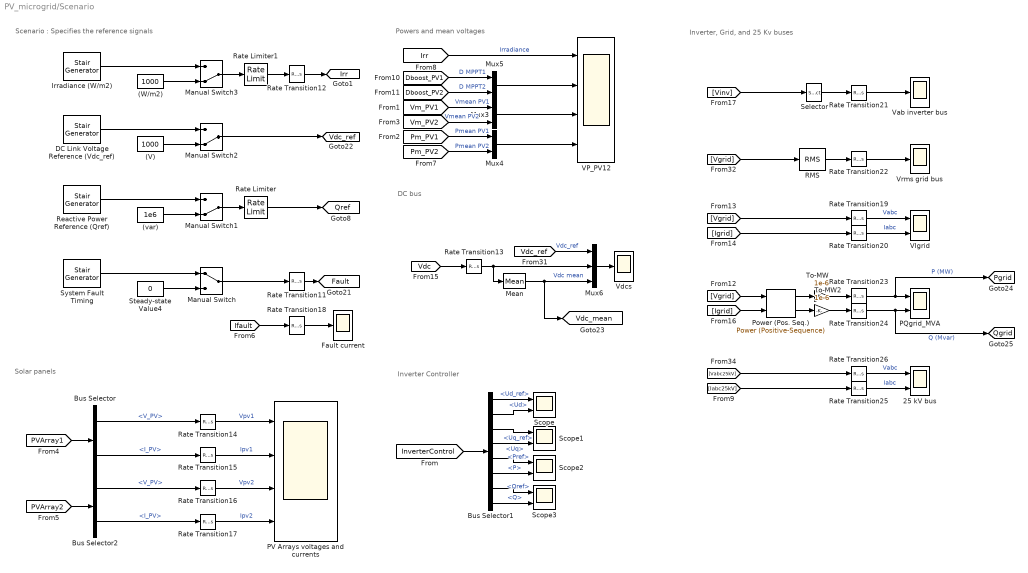
== system PV_microgrid/Scenario ==
  note: DC bus
  note: Powers and mean voltages
  note: Inverter, Grid, and 25 Kv buses
  note: Inverter Controller
  note: Solar panels
  note: Scenario : Specifies the reference signals
  (V) : Constant  Value=1000
  (W/m2) : Constant  Value=1000
  (var) : Constant  Value=1e6
  25 kV bus : Scope  NumInputPorts=2
  Bus Selector : BusSelector  OutputSignals=V_PV,I_PV
  Bus Selector1 : BusSelector  OutputSignals=Ud_ref,Ud,Uq_ref,Uq,Pref,P,Qref,Q
  Bus Selector2 : BusSelector  OutputSignals=V_PV,I_PV
  DC Link Voltage Reference (Vdc_ref) : spsStairGeneratorLib/Stair Generator  t=[0, 0.2, 0.4]  e=[1000, 1050, 1000]  Ts=Ts
  Fault current : Scope
  Irradiance (W/m2) : spsStairGeneratorLib/Stair Generator  t=[0, 0.2, 0.4]  e=[1000, 250,1000]  Ts=Ts
  Manual Switch : ManualSwitch
  Manual Switch1 : ManualSwitch  CurrentSetting=0
  Manual Switch2 : ManualSwitch  CurrentSetting=0
  Manual Switch3 : ManualSwitch  CurrentSetting=0
  Mean : spsMeanLib/Mean  Freq=60  Vinit=1000  Ts=Ts
  Mux3 : Mux  Inputs=2
  Mux4 : Mux  Inputs=2
  Mux5 : Mux  Inputs=2
  Mux6 : Mux  Inputs=3
  PQgrid_MVA : Scope  NumInputPorts=2
  PV Arrays voltages and currents : Scope  NumInputPorts=4
  Power (Pos. Seq.) : spsPowerPositiveSequenceLib/Power (Positive-Sequence)  Freq=50  Vinit=[20570,-37]  Iinit=[70, -63]  Ts=Ts_Power
      settings: LibrarySourceBlock=|
      | sps_lib/Sensors and Measurements/Power
      | (Positive-Sequence)
  RMS : spsRMSLib/RMS  TrueRMS=off  Freq=50  RMSInit=25000  Ts=Ts_Power
  Rate Limiter : RateLimiter  RisingSlewLimit=1e6/(1/60)  FallingSlewLimit=-1e6/(1/60)  SampleTimeMode=inherited  InitialCondition=1e6
  Rate Limiter1 : RateLimiter  RisingSlewLimit=1000/(1/60)  FallingSlewLimit=-1000/(1/60)  SampleTimeMode=inherited  InitialCondition=1000
  Rate Transition11 : RateTransition  OutPortSampleTime=Ts_Power
  Rate Transition12 : RateTransition  OutPortSampleTime=Ts_Power
  Rate Transition{13..26} (14 alike) : RateTransition  OutPortSampleTime=Ts
  "Reactive Power Reference (Qref) " : spsStairGeneratorLib/Stair Generator  t=[0, 0.2, 0.4]  e=[1e6, -1e6, 1e6]  Ts=Ts
  Scope{,1..3} (4 alike) : Scope  NumInputPorts=2
  Selector : Selector  InputPortWidth=3  IndexOptions=Index vector (dialog)  Indices=1  OutputSizes=1
  Steady-state Value4 : Constant  Value=0
  System Fault Timing : spsStairGeneratorLib/Stair Generator  t=[0, 0.25, 0.45]  e=[0, 1, 0]  Ts=Ts
  To-MW : Gain  Gain=1e-6
  To-MW2 : Gain  Gain=1e-6
  VIgrid : Scope  NumInputPorts=2
  VP_PV12 : Scope  NumInputPorts=4
  Vab inverter bus : Scope
  Vdcs : Scope
  Vrms grid bus : Scope
  tag scope: Fault=global, Irr=global, Pgrid=global, Qgrid=global, Qref=global, Vdc_mean=global, Vdc_ref=global
  wires:
  Rate Limiter/1 -> [Qref]
  (W/m2)/1 -> Manual Switch3/2
  (V)/1 -> Manual Switch2/2
  Steady-state Value4/1 -> Manual Switch/2
  DC Link Voltage Reference (Vdc_ref)/1 -> Manual Switch2/1
  System Fault Timing/1 -> Manual Switch/1
  Manual Switch/1 -> Rate Transition11/1
  Rate Limiter1/1 -> Rate Transition12/1
  (var)/1 -> Manual Switch1/2
  "Reactive Power Reference (Qref) "/1 -> Manual Switch1/1
  Manual Switch1/1 -> Rate Limiter/1
  Manual Switch2/1 -> [Vdc_ref]
  Irradiance (W/m2)/1 -> Manual Switch3/1
  Manual Switch3/1 -> Rate Limiter1/1
  Rate Transition12/1 -> [Irr]
  Bus Selector2/1 -> Rate Transition16/1  "<V_PV>"
  Bus Selector/2 -> Rate Transition15/1  "<I_PV>"
  Bus Selector/1 -> Rate Transition14/1  "<V_PV>"
  Rate Transition19/1 -> VIgrid/1  "Vabc"
  [Pm_PV1] -> Mux4/1  "Pmean PV1"
  Rate Transition17/1 -> PV Arrays voltages and currents/4  "Ipv2"
  RMS/1 -> Rate Transition22/1
  [Pm_PV2] -> Mux4/2  "Pmean PV2"
  [Irr] -> VP_PV12/1  "Irradiance"
  Rate Transition22/1 -> Vrms grid bus/1
  Rate Transition16/1 -> PV Arrays voltages and currents/3  "Vpv2"
  Rate Transition26/1 -> 25 kV bus/1  "Vabc"
  Mux3/1 -> VP_PV12/3
  [Vgrid] -> RMS/1
  [Vgrid] -> Power (Pos. Seq.)/1
  Rate Transition23/1 -> [Pgrid], PQgrid_MVA/1  "P (MW)"
  [PVArray1] -> Bus Selector/1
  Rate Transition20/1 -> VIgrid/2  "Iabc"
  Mux6/1 -> Vdcs/1
  Mux4/1 -> VP_PV12/4
  Rate Transition15/1 -> PV Arrays voltages and currents/2  "Ipv1"
  Mux5/1 -> VP_PV12/2
  Power (Pos. Seq.)/2 -> To-MW2/1
  [Igrid] -> Rate Transition20/1
  Rate Transition18/1 -> Fault current/1
  [Vabc25kV] -> Rate Transition26/1
  Rate Transition25/1 -> 25 kV bus/2  "Iabc"
  [Vm_PV2] -> Mux3/2  "Vmean PV2"
  Rate Transition14/1 -> PV Arrays voltages and currents/1  "Vpv1"
  [Vgrid] -> Rate Transition19/1
  Rate Transition13/1 -> Mean/1, Mux6/2
  Power (Pos. Seq.)/1 -> To-MW/1
  [Dboost_PV1] -> Mux5/1  "D MPPT1"
  [Vinv] -> Selector/1
  Mean/1 -> Mux6/3, [Vdc_mean]  "Vdc mean"
  Rate Transition11/1 -> [Fault]
  [Dboost_PV2] -> Mux5/2  "D MPPT2"
  [Vm_PV1] -> Mux3/1  "Vmean PV1"
  [Vdc_ref] -> Mux6/1  "Vdc_ref"
  [Igrid] -> Power (Pos. Seq.)/2
  Bus Selector2/2 -> Rate Transition17/1  "<I_PV>"
  [Iabc25kV] -> Rate Transition25/1
  Rate Transition24/1 -> [Qgrid], PQgrid_MVA/2  "Q (Mvar)"
  [Vdc] -> Rate Transition13/1
  [PVArray2] -> Bus Selector2/1
  [Ifault] -> Rate Transition18/1
  Selector/1 -> Rate Transition21/1
  Rate Transition21/1 -> Vab inverter bus/1
  To-MW2/1 -> Rate Transition24/1
  To-MW/1 -> Rate Transition23/1
  [InverterControl] -> Bus Selector1/1
  Bus Selector1/1 -> Scope/1  "<Ud_ref>"
  Bus Selector1/2 -> Scope/2  "<Ud>"
  Bus Selector1/3 -> Scope1/1  "<Uq_ref>"
  Bus Selector1/4 -> Scope1/2  "<Uq>"
  Bus Selector1/8 -> Scope3/2  "<Q>"
  Bus Selector1/7 -> Scope3/1  "<Qref>"
  Bus Selector1/6 -> Scope2/2  "<P>"
  Bus Selector1/5 -> Scope2/1  "<Pref>"

== system PV_microgrid/Subsystem1 ==

== system PV_microgrid/Subsystem2 ==

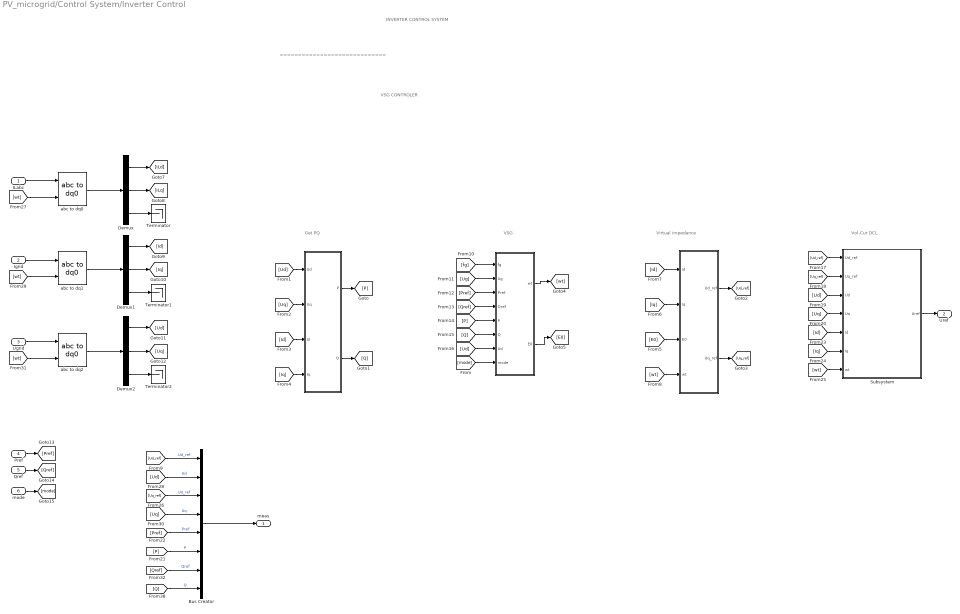
== system PV_microgrid/Control System/Inverter Control ==
  note: INVERTER CONTROL SYSTEM
  note: =============================
  note: VSG
  note: Vol-Cur DCL
  note: Get PQ
  note: Virtual impedance
  note: VSG CONTROLER
  ILabc : Inport
  Igrid : Inport  Port=2
  Ugrid : Inport  Port=3
  Pref : Inport  Port=4
  Qref : Inport  Port=5
  mode : Inport  Port=6
  " " : Subsystem
  "  " : Subsystem
  "   " : Subsystem
  Bus Creator : BusCreator  Inputs=8
  Demux : Demux  Outputs=3
  Demux1 : Demux  Outputs=3
  Demux2 : Demux  Outputs=3
  Subsystem : Subsystem
  Terminator : Terminator
  Terminator1 : Terminator
  Terminator2 : Terminator
  abc to dq0 : spsabctodq0Lib/abc to dq0  Alignment=90 degrees behind phase A axis
  abc to dq1 : spsabctodq0Lib/abc to dq0  Alignment=90 degrees behind phase A axis
  abc to dq2 : spsabctodq0Lib/abc to dq0  Alignment=90 degrees behind phase A axis
  meas : Outport  VectorParamsAs1DForOutWhenUnconnected=off
  Uref : Outport  Port=2
  wires:
  [Iq] -> " "/4(Iq)
  [Iq] -> Subsystem/6(Iq)
  "  "/1(wt) -> [wt]
  Subsystem/1(Uref) -> Uref/1
  [P] -> "  "/5(P)
  [wt] -> Subsystem/7(wt)
  ILabc/1 -> abc to dq0/1
  Demux2/3 -> Terminator2/1
  [Ud] -> " "/1(Ud)
  [Qref] -> "  "/4(Qref)
  Demux2/2 -> [Uq]
  [Ud] -> Subsystem/3(Ud)
  [Q] -> "  "/6(Q)
  [Pref] -> "  "/3(Pref)
  [wt] -> abc to dq2/2
  "   "/1(Ud_ref) -> [Ud_ref]
  abc to dq2/1 -> Demux2/1
  [Id] -> Subsystem/5(Id)
  Demux/3 -> Terminator/1
  [Ug] -> "  "/2(Ug)
  [wt] -> abc to dq0/2
  [Ud_ref] -> Subsystem/1(Ud_ref)
  abc to dq1/1 -> Demux1/1
  [Uq] -> Subsystem/4(Uq)
  abc to dq0/1 -> Demux/1
  Demux1/1 -> [Id]
  Demux1/2 -> [Iq]
  Demux/2 -> [ILq]
  " "/1(P) -> [P]
  Demux/1 -> [ILd]
  Demux2/1 -> [Ud]
  [Uq_ref] -> Subsystem/2(Uq_ref)
  "   "/2(Uq_ref) -> [Uq_ref]
  " "/2(Q) -> [Q]
  [Uq] -> " "/2(Uq)
  "  "/2(E0) -> [E0]
  [Id] -> " "/3(Id)
  [Id] -> "   "/1(Id)
  [fg] -> "  "/1(fg)
  Demux1/3 -> Terminator1/1
  [Iq] -> "   "/2(Iq)
  [wt] -> abc to dq1/2
  Ugrid/1 -> abc to dq2/1
  [wt] -> "   "/4(wt)
  Igrid/1 -> abc to dq1/1
  [E0] -> "   "/3(E0)
  [Ud] -> "  "/7(Ud)
  [Qref] -> Bus Creator/7  "Qref"
  [P] -> Bus Creator/6  "P"
  Bus Creator/1 -> meas/1
  [Pref] -> Bus Creator/5  "Pref"
  [mode] -> "  "/8(mode)
  [Uq] -> Bus Creator/4  "Uq"
  [Uq_ref] -> Bus Creator/3  "Uq_ref"
  [Ud] -> Bus Creator/2  "Ud"
  Pref/1 -> [Pref]
  Qref/1 -> [Qref]
  mode/1 -> [mode]
  [Ud_ref] -> Bus Creator/1  "Ud_ref"
  [Q] -> Bus Creator/8  "Q"

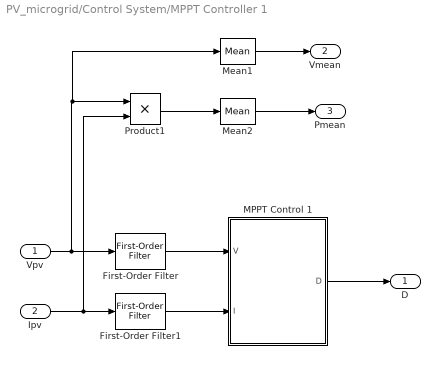
== system PV_microgrid/Control System/MPPT Controller 1 ==
  Vpv : Inport
  Ipv : Inport  Port=2
  First-Order Filter : spsFirstOrderFilterLib/First-Order Filter  FilterType=Lowpass  Tc=1/Fc  Ts=Ts  Initialize=off  Vac_Init=[0, 0, 60]  Vdc_Init=0  PlotResponse=off  FreqRange="[0,  200,  1]"
  First-Order Filter1 : spsFirstOrderFilterLib/First-Order Filter  FilterType=Lowpass  Tc=1/Fc  Ts=Ts  Initialize=off  Vac_Init=[0, 0, 60]  Vdc_Init=0  PlotResponse=off  FreqRange="[0,  200,  1]"
  "MPPT Control 1 " : MATLAB Function  TreatAsAtomicUnit=on
  Mean1 : spsMeanLib/Mean  Freq=60  Vinit=650  Ts=Ts
  Mean2 : spsMeanLib/Mean  Freq=60  Vinit=1500e3  Ts=Ts
  Product1 : Product
  D : Outport  VectorParamsAs1DForOutWhenUnconnected=off
  Vmean : Outport  Port=2  VectorParamsAs1DForOutWhenUnconnected=off
  Pmean : Outport  Port=3  VectorParamsAs1DForOutWhenUnconnected=off
  wires:
  First-Order Filter1/1 -> "MPPT Control 1 "/2(I)
  First-Order Filter/1 -> "MPPT Control 1 "/1(V)
  Ipv/1 -> Product1/2, First-Order Filter1/1
  Vpv/1 -> Mean1/1, Product1/1, First-Order Filter/1
  "MPPT Control 1 "/1(D) -> D/1
  Product1/1 -> Mean2/1
  Mean1/1 -> Vmean/1
  Mean2/1 -> Pmean/1

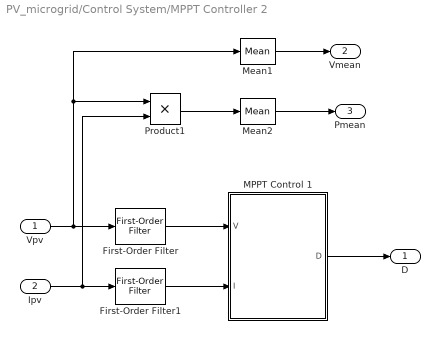
== system PV_microgrid/Control System/MPPT Controller 2 ==
  Vpv : Inport
  Ipv : Inport  Port=2
  First-Order Filter : spsFirstOrderFilterLib/First-Order Filter  FilterType=Lowpass  Tc=1/Fc  Ts=Ts  Initialize=off  Vac_Init=[0, 0, 60]  Vdc_Init=0  PlotResponse=off  FreqRange="[0,  200,  1]"
  First-Order Filter1 : spsFirstOrderFilterLib/First-Order Filter  FilterType=Lowpass  Tc=1/Fc  Ts=Ts  Initialize=off  Vac_Init=[0, 0, 60]  Vdc_Init=0  PlotResponse=off  FreqRange="[0,  200,  1]"
  "MPPT Control 1 " : MATLAB Function  TreatAsAtomicUnit=on
  Mean1 : spsMeanLib/Mean  Freq=60  Vinit=420  Ts=Ts
  Mean2 : spsMeanLib/Mean  Freq=60  Vinit=500e3  Ts=Ts
  Product1 : Product
  D : Outport  VectorParamsAs1DForOutWhenUnconnected=off
  Vmean : Outport  Port=2  VectorParamsAs1DForOutWhenUnconnected=off
  Pmean : Outport  Port=3  VectorParamsAs1DForOutWhenUnconnected=off
  wires:
  "MPPT Control 1 "/1(D) -> D/1
  Ipv/1 -> Product1/2, First-Order Filter1/1
  First-Order Filter/1 -> "MPPT Control 1 "/1(V)
  First-Order Filter1/1 -> "MPPT Control 1 "/2(I)
  Mean1/1 -> Vmean/1
  Product1/1 -> Mean2/1
  Mean2/1 -> Pmean/1
  Vpv/1 -> Product1/1, Mean1/1, First-Order Filter/1

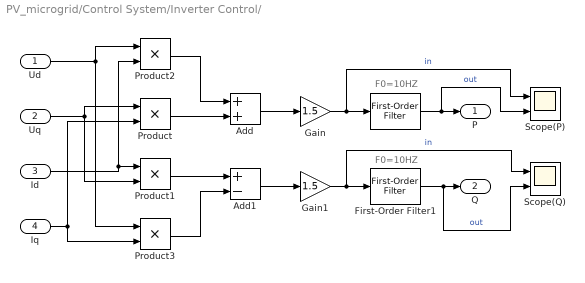
== system PV_microgrid/Control System/Inverter Control/  ==
  note: F0=10HZ
  note: F0=10HZ
  Ud : Inport
  Uq : Inport  Port=2
  Id : Inport  Port=3
  Iq : Inport  Port=4
  " " : spsFirstOrderFilterLib/First-Order Filter  FilterType=Lowpass  Tc=10e-3  Ts=1/fsw  Initialize=on  Vac_Init=[0, 0, 10]  Vdc_Init=0  PlotResponse=off  FreqRange="[0,  200,  1]"
  Add : Sum
  Add1 : Sum  Inputs=+-
  First-Order Filter1 : spsFirstOrderFilterLib/First-Order Filter  FilterType=Lowpass  Tc=10e-3  Ts=1/fsw  Initialize=on  Vac_Init=[0, 0, 10]  Vdc_Init=0  PlotResponse=off  FreqRange="[0,  200,  1]"
  Gain : Gain  Gain=1.5
  Gain1 : Gain  Gain=1.5
  Product{,1..3} (4 alike) : Product
  Scope(P) : Scope  NumInputPorts=2
  Scope(Q) : Scope  NumInputPorts=2
  P : Outport
  Q : Outport  Port=2
  wires:
  Gain1/1 -> First-Order Filter1/1, Scope(Q)/1  "in"
  Product2/1 -> Add/1
  " "/1 -> Scope(P)/2, P/1  "out"
  Add1/1 -> Gain1/1
  Gain/1 -> " "/1, Scope(P)/1  "in"
  First-Order Filter1/1 -> Scope(Q)/2, Q/1  "out"
  Product/1 -> Add/2
  Product3/1 -> Add1/2
  Product1/1 -> Add1/1
  Ud/1 -> Product3/1, Product2/1
  Add/1 -> Gain/1
  Id/1 -> Product1/1, Product2/2
  Iq/1 -> Product3/2, Product/2
  Uq/1 -> Product1/2, Product/1
